simulink model "Flujo_Anticipativo"  (R2019a)
settings: Solver=VariableStepAuto  StartTime=0.0  StopTime=150  RelTol=1e-3
values from neighbouring files (symbols this model uses):
  Dfd = [8.12426970428 24.4353933777 34.4322603162 28.1505552728 13.4873533711 3.31175732259 0.248550757084]    [DatosDF.mat]
  Dff = [1 4.2492917847 8.42635764672 9.54828061951 6.08601455918 1.72408344453]    [DatosDF.mat]
  DGcc = [5.21016271128 49.2173016974 214.486679616 563.108464374 834.214301772 697.431084229 217.165994152 22.4570540102 0.246049619203]    [DatosPF.mat]
  DGp = [5.21016271128 47.7445548362 204.683846511 505.80083821 720.009966666 497.843847616 72.3392867678]    [DatosPF.mat]
  Nfd = [0 -0.0125032287598 0.0360670060378 -0.048551738897 0.0373474914592 -0.016159972266 0.00310768697423]    [DatosDF.mat]
  Nff = [-1 4.2492917847 -8.42635764672 9.54828061951 -6.08601455918 1.72408344453]    [DatosDF.mat]
  NGcc = [68.0968266364 679.916650227 3195.64641265 8882.00560393 15159.700912 15029.0411187 7422.16617011 1561.37333599 114.109293055]    [DatosPF.mat]
  NGp = [0 -0.0170151807 0.152656853798 -0.639150054516 1.52915427931 -2.05789070389 1.23086603606]    [DatosPF.mat]
settings Model: Creator=Exilo  LastModifiedBy=Exilo

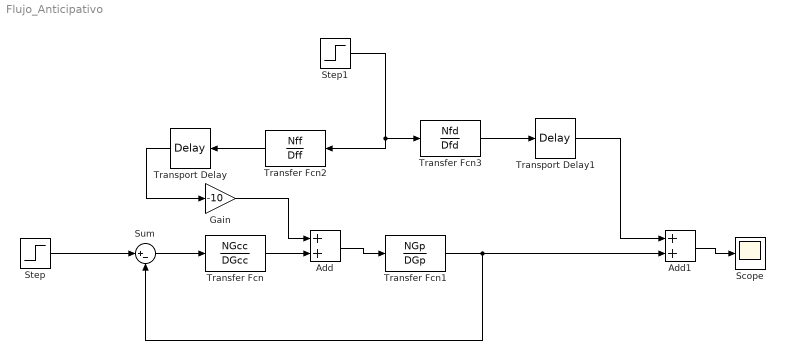
== system Flujo_Anticipativo ==
  Add : Sum
  Add1 : Sum
  Gain : Gain  Gain=-10
  Scope : Scope
  Step : Step  Before=10000  After=27000  SampleTime=0
  Step1 : Step  Before=15000  After=20000  SampleTime=0
  Sum : Sum  Inputs=|+-
  Transfer Fcn : TransferFcn  Numerator=NGcc  Denominator=DGcc
  Transfer Fcn1 : TransferFcn  Numerator=NGp  Denominator=DGp
  Transfer Fcn2 : TransferFcn  Numerator=Nff  Denominator=Dff
  Transfer Fcn3 : TransferFcn  Numerator=Nfd  Denominator=Dfd
  Transport Delay : TransportDelay  DelayTime=60
  Transport Delay1 : TransportDelay  DelayTime=60
  wires:
  Step/1 -> Sum/1
  Sum/1 -> Transfer Fcn/1
  Transfer Fcn1/1 -> Add1/2, Sum/2
  Transfer Fcn/1 -> Add/2
  Add/1 -> Transfer Fcn1/1
  Transfer Fcn2/1 -> Transport Delay/1
  Transfer Fcn3/1 -> Transport Delay1/1
  Step1/1 -> Transfer Fcn2/1, Transfer Fcn3/1
  Add1/1 -> Scope/1
  Transport Delay/1 -> Gain/1
  Transport Delay1/1 -> Add1/1
  Gain/1 -> Add/1
